simulink model "ex7_custom_block"  (R2022a)
settings: Solver=VariableStepAuto  StartTime=0.0  StopTime=0.1  RelTol=1e-3
values from neighbouring files (symbols this model uses):
  Rb = 100e3    (= 100000)    [ex6_parameters.m]
libraries: commsink2 x1, commrandsrc3 x1
settings Model: Creator=Filippo  LastModifiedBy=Filippo

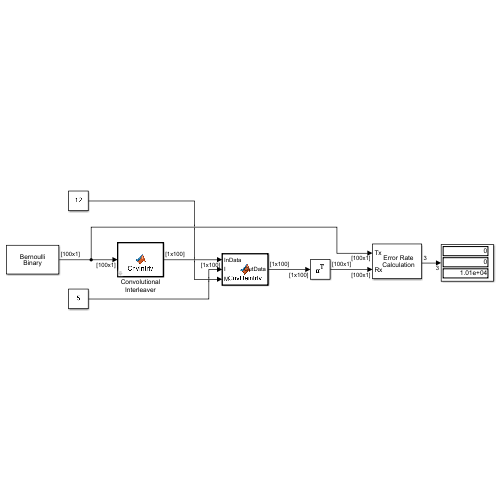
[thumbnail: Simulink's stored preview of the top-level diagram]
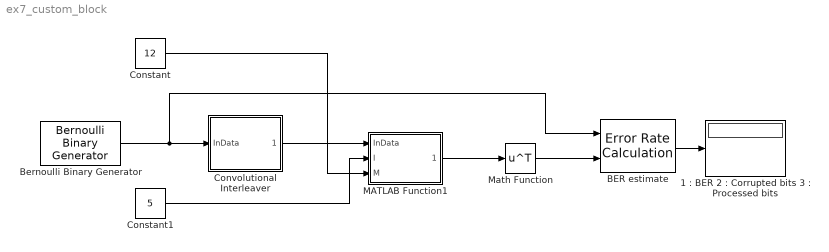
== system ex7_custom_block ==
  "1 : BER 2 : Corrupted bits 3 : Processed bits" : Display
  BER estimate : commsink2/Error Rate Calculation  N=0  st_delay=0  cp_mode=Entire frame  subframe=[]  PMode=Port  WsName=ErrorVec  RsMode2=off  stop=off  numErr=100  maxBits=1e6
  Bernoulli Binary Generator : commrandsrc3/Bernoulli Binary Generator  ProbabilityOfZero=0.5  SeedSource=Auto  Seed=0  SampleTime=1/Rb  SamplesPerFrame=100  OutputDataType=uint8  SimulateUsing=Interpreted execution
  Constant : Constant  Value=12
  Constant1 : Constant  Value=5
  Convolutional Interleaver : MATLAB Function  TreatAsAtomicUnit=on  mask{I=5, M=12}
      mask prompts: I "Number of delay lines (I)"; M "Number of delay cells per block (M)"
  MATLAB Function1 : MATLAB Function  TreatAsAtomicUnit=on
  Math Function : Math  Operator=transpose
  wires:
  Bernoulli Binary Generator/1 -> Convolutional Interleaver/1(InData), BER estimate/1
  Constant1/1 -> MATLAB Function1/2(I)
  BER estimate/1 -> "1 : BER 2 : Corrupted bits 3 : Processed bits"/1
  MATLAB Function1/1(OutData) -> Math Function/1
  Math Function/1 -> BER estimate/2
  Constant/1 -> MATLAB Function1/3(M)
  Convolutional Interleaver/1(OutData) -> MATLAB Function1/1(InData)

== matlab function ex7_custom_block/MATLAB Function1 ==
  data: InData input; OutData output; I input; M input

% >> Function for implementing a convolutional deinterleaver. It requires as input the data
%    vector and the number of delay lines (I) and the number of delay cells per block (M). 
function OutData   = CnvDeintrlv( InData, I, M )
    Len = length(InData);                                                           % overall I/O buffers length
    OutData = uint8(zeros(1,Len));
    ShReg = NaN(I-1,M*(I-1));                                                       % shift register matrix (NaN means the cell is empty)
    InIdx = 1;                                                                      % index over input array
    OutIdx = 1;                                                                     % index over output array
    RwIdx = 1;                                                                      % row index
    ClIdx = 0;                                                                      % column index (-1)
    while OutIdx <= Len 
        if RwIdx == I && RwIdx+I*(ClIdx-M*(RwIdx-1)) <= Len
            OutData(OutIdx) = InData(InIdx);                                        % output from no-delay line
            OutIdx = OutIdx+1;
            InIdx = InIdx+1;
        else
            if ~(isnan(ShReg(RwIdx,M*(I-RwIdx))))
                OutData(OutIdx) = ShReg(RwIdx,M*(I-RwIdx));                         % output from shift registers
                OutIdx = OutIdx+1;
            end
            for j = M*(I-RwIdx):-1:2
                ShReg(RwIdx,j) = ShReg(RwIdx,j-1);                                  % update shift-registers (by right-shifting)
            end
            if RwIdx+I*(ClIdx-M*(RwIdx-1)) <= Len
                ShReg(RwIdx,1) = InData(InIdx);
                InIdx = InIdx+1;
            else
                ShReg(RwIdx,1) = NaN;
            end
        end
        if ClIdx < M*(I-1)                                                          % case for 1st phase (initial transient)
            if RwIdx == floor(ClIdx/M)+1                                            % "floor" is for executing the operation of integer-division
                RwIdx = 1;
                ClIdx = ClIdx+1;
            else
                RwIdx = RwIdx+1;
            end
        else                                                                        % case for 2nd phase (shift-registers filled)
            if RwIdx == I
                RwIdx = 1;
                ClIdx = ClIdx+1;
            else
                RwIdx = RwIdx+1;
            end
        end
    end
end

== matlab function ex7_custom_block/Convolutional Interleaver ==
  data: InData input; OutData output; M parameter; I parameter

% >> Function for implementing a convolutional interleaver. It requires as the data vector
%    and the number of delay lines (I) and the number of delay cells per block (M). 
function OutData = CnvIntrlv( InData, M,  I)
    Len = length(InData);                                                           % overall I/O buffers length
    OutData = uint8(zeros(1,Len));
    ShReg = NaN(I-1,M*(I-1));                                                       % shift register matrix (NaN means the cell is empty)
    InIdx = 1;                                                                      % index over input array
    OutIdx = 1;                                                                     % index over output array
    RwIdx = 0;                                                                      % row index ("0" represents the line with no delay)
    while InIdx <= Len                                                              % loop until all input elements are consumed...
        if RwIdx == 0
            OutData(OutIdx) = InData(InIdx);                                        % output from no-delay line
            OutIdx = OutIdx+1;
        else 
            if ~(isnan(ShReg(RwIdx,M*RwIdx)))
                OutData(OutIdx) = ShReg(RwIdx,M*RwIdx);                             % output from shift-registers
                OutIdx = OutIdx+1;
            end
            for j = M*(RwIdx):-1:2
                ShReg(RwIdx,j) = ShReg(RwIdx,j-1);                                  % update shift-registers (by right-shifting)
            end
            ShReg(RwIdx,1) = InData(InIdx);
        end
        InIdx = InIdx+1;
        
        if RwIdx == I-1
            RwIdx = 0;
        else
            RwIdx = RwIdx+1;
        end
    end
    if RwIdx == 0
        RwIdx = 1;
    end
    while OutIdx <= Len                                                             % loop until all elements still stored in the shift-register has been completely consumed...
        if ~(isnan(ShReg(RwIdx,M*RwIdx)))
            OutData(OutIdx) = ShReg(RwIdx,M*RwIdx);
            OutIdx = OutIdx+1;
        end
        for j = M*(RwIdx):-1:2
            ShReg(RwIdx,j) = ShReg(RwIdx,j-1);
        end
        ShReg(RwIdx,1) = NaN;
        if RwIdx == I-1
            RwIdx = 1;
        else
            RwIdx = RwIdx+1;
        end
    end
end
